simulink model "untitled"  (R2022b)
settings: Solver=ode4  StartTime=0.0  StopTime=500  FixedStep=10  RelTol=1e-3
settings Model: Creator=asus  LastModifiedBy=asus

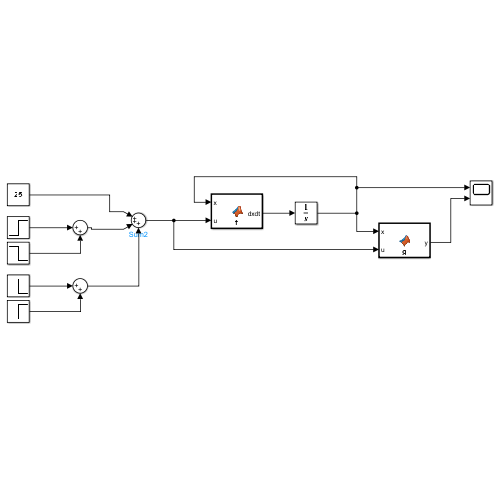
[thumbnail: Simulink's stored preview of the top-level diagram]
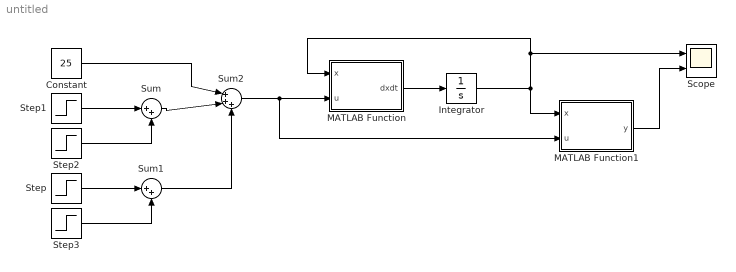
== system untitled ==
  Constant : Constant  Value=25
  Integrator : Integrator  InitialCondition=[0 ; 0 ; 0]
  MATLAB Function : MATLAB Function  TreatAsAtomicUnit=on
  MATLAB Function1 : MATLAB Function  TreatAsAtomicUnit=on
  Scope : Scope  NumInputPorts=2
  Step : Step  Time=300  After=-5  SampleTime=0
  Step1 : Step  Time=100  After=5  SampleTime=0
  Step2 : Step  Time=200  After=-5  SampleTime=0
  Step3 : Step  Time=400  After=5  SampleTime=0
  Sum : Sum  Inputs=|++
  Sum1 : Sum  Inputs=|++
  Sum2 : Sum  Inputs=|+++
  wires:
  Sum1/1 -> Sum2/3
  Sum2/1 -> MATLAB Function1/2(u), MATLAB Function/2(u)
  Step1/1 -> Sum/1
  Integrator/1 -> Scope/1, MATLAB Function/1(x), MATLAB Function1/1(x)
  Sum/1 -> Sum2/2
  Step/1 -> Sum1/1
  Step3/1 -> Sum1/2
  MATLAB Function1/1(y) -> Scope/2
  Constant/1 -> Sum2/1
  MATLAB Function/1(dxdt) -> Integrator/1
  Step2/1 -> Sum/2

== matlab function untitled/MATLAB Function ==
  data: x input; u input; dxdt output
function dxdt = f(x, u)
    M = 0.48*(1-0.02*x(3))*x(2) / (1.2+x(2)+(x(2)^2)/22);
    dxdt = [-0.15*x(1) + M*x(1);
            0.15*(u-x(2))-2.5*M*x(1);
            -0.15*x(3)+(2.2*M+0.2)*x(1)];
end

== matlab function untitled/MATLAB Function1 ==
  data: x input; u input; y output
function y = g(x, u)
    y = x(3);
end
